simulink model "IMU"  (R2018a)
settings: Solver=VariableStepAuto  StartTime=0.0  StopTime=10.0  RelTol=1e-3
libraries: sensors x3
settings Model: Creator=David  LastModifiedBy=David

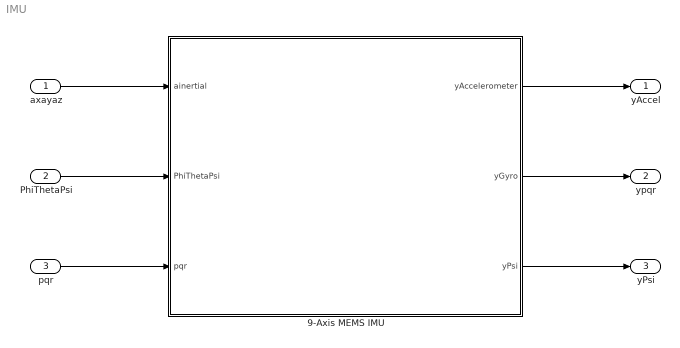
== system IMU ==
  axayaz : Inport
  PhiThetaPsi : Inport  Port=2
  pqr : Inport  Port=3
  9-Axis MEMS IMU : Subsystem
      mask Display:
      | image('VNAV_IMU.jpg')
      | 
      | color('green')
      | 
      | port_label('input', 1, '{\bfa_{inertial}} (m/s^2)', 'texMode', 'on')
      | port_label('input', 2, '[\phi, \theta, \psi] (rad)', 'texMode', 'on')
      | port_label('input', 3, '{\bf\omega_b} (rad/s)', 'texMode', 'on')
      | 
      | port_label('output', 1, '[y_{accel_x}, y_{accel_y}, y_{accel_z}] (m/s^2)', 'texMode', 'on')
      | port_label('output', 2, '[y_p, y_q, y_r] (rad/s)', 'texMode', 'on')
      | port_label('output', 3, 'y_{\psi} (rad)', 'texMode', 'on')
  yAccel : Outport
  ypqr : Outport  Port=2
  yPsi : Outport  Port=3
  wires:
  9-Axis MEMS IMU/1(yAccelerometer) -> yAccel/1
  9-Axis MEMS IMU/2(yGyro) -> ypqr/1
  9-Axis MEMS IMU/3(yPsi) -> yPsi/1
  axayaz/1 -> 9-Axis MEMS IMU/1(ainertial)
  PhiThetaPsi/1 -> 9-Axis MEMS IMU/2(PhiThetaPsi)
  pqr/1 -> 9-Axis MEMS IMU/3(pqr)

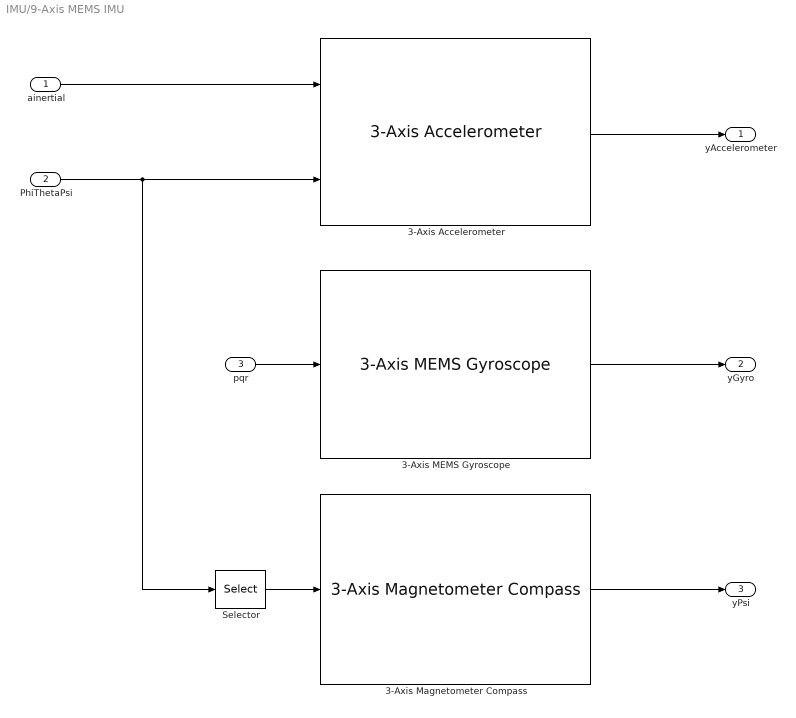
== system IMU/9-Axis MEMS IMU ==
  ainertial : Inport
  PhiThetaPsi : Inport  Port=2
  pqr : Inport  Port=3
  3-Axis Accelerometer : sensors/3-Axis Accelerometer  g=9.81  SampleTime=0.01  accelXNoiseDensity=0.1/sqrt(100)  accelYNoiseDensity=0.1/sqrt(100)  accelZNoiseDensity=0.1/sqrt(100)  accelXBandwidthHz=1000  accelYBandwidthHz=1000  accelZBandwidthHz=1000  accelXInit=0  accelYInit=0  accelZInit=0  accelXUpperSaturation=inf  accelXLowerSaturation=-inf  accelYUpperSaturation=inf  accelYLowerSaturation=-inf  accelZUpperSaturation=inf  accelZLowerSaturation=-inf  accelXResolution=1E-12  accelYResolution=1E-12  accelZResolution=1E-12
  3-Axis MEMS Gyroscope : sensors/3-Axis MEMS Gyroscope  SampleTime=0.01  gyroXNoiseDensity=0  gyroYNoiseDensity=0  gyroZNoiseDensity=0  gyroXBandwidthHz=1E06  gyroYBandwidthHz=1E06  gyroZBandwidthHz=1E06  gyroXInit=0  gyroYInit=0  gyroZInit=0  gyroXUpperSaturation=inf  gyroXLowerSaturation=-inf  gyroYUpperSaturation=inf  gyroYLowerSaturation=-inf  gyroZUpperSaturation=inf  gyroZLowerSaturation=-inf  gyroXResolution=1E-06  gyroYResolution=1E-06  gyroZResolution=1E-06
  3-Axis Magnetometer Compass : sensors/3-Axis Magnetometer Compass  SampleTime=1  headingNoiseDensity=0  headingBandwidthHz=1E06  headingInit=0  headingUpperSaturation=inf  headingLowerSaturation=-inf  headingResolution=1E-06
  Selector : Selector  InputPortWidth=3  IndexOptions=Index vector (dialog)  Indices=3  OutputSizes=1
  yAccelerometer : Outport
  yGyro : Outport  Port=2
  yPsi : Outport  Port=3
  wires:
  ainertial/1 -> 3-Axis Accelerometer/1
  PhiThetaPsi/1 -> 3-Axis Accelerometer/2, Selector/1
  Selector/1 -> 3-Axis Magnetometer Compass/1
  pqr/1 -> 3-Axis MEMS Gyroscope/1
  3-Axis MEMS Gyroscope/1 -> yGyro/1
  3-Axis Accelerometer/1 -> yAccelerometer/1
  3-Axis Magnetometer Compass/1 -> yPsi/1
